simulink model "PTSD_single_channel_local_min_max"  (R2019b)
settings: Solver=VariableStepAuto  StartTime=0.0  StopTime=10  RelTol=1e-3
libraries: simulink x4, dspswit3 x1
settings Model: Creator=sbuccelli  LastModifiedBy=sbuccelli

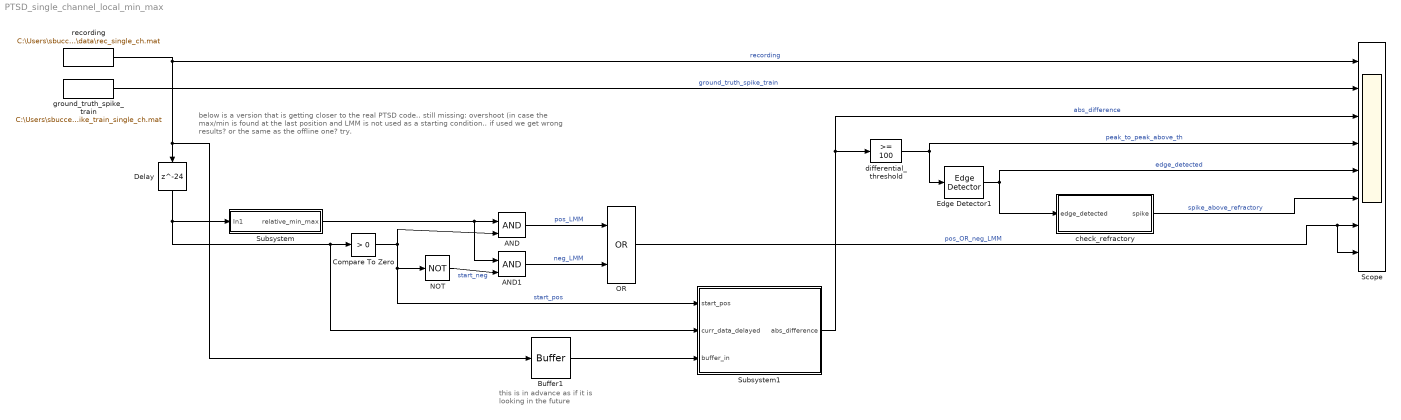
== system PTSD_single_channel_local_min_max ==
  note: below is a version that is getting closer to the real PTSD code..
      | still missing: overshoot (in case the max/min is found at the last position and LMM is not used as a starting condition.. if used we get wrong results? or the same as the offline one? try.
  note: this is in advance as if it is looking in the future
  AND : Logic  IconShape=distinctive  AllPortsSameDT=off  OutDataTypeStr=boolean
  AND1 : Logic  IconShape=distinctive  AllPortsSameDT=off  OutDataTypeStr=boolean
  Buffer1 : Buffer  N=24  V=23  OutputFrames=off
  Compare To Zero : simulink/Logic and Bit Operations/Compare To Zero  relop=>  OutDataTypeStr=boolean
  Delay : Delay  DelayLength=24
  Edge Detector1 : dspswit3/Edge Detector  InputProcessing=Columns as channels (frame based)
      settings: SourceProductName=DSP System Toolbox  SourceProductBaseCode=DS
  NOT : Logic  Operator=NOT  IconShape=distinctive  AllPortsSameDT=off  OutDataTypeStr=boolean
  OR : Logic  Operator=OR  IconShape=distinctive  AllPortsSameDT=off  OutDataTypeStr=boolean
  Scope : Scope  NumInputPorts=8
  Subsystem : Subsystem
  Subsystem1 : Subsystem
  check_refractory : Subsystem
  differential_threshold : simulink/Logic and Bit Operations/Compare To Constant  relop=>=  const=100  OutDataTypeStr=boolean
  ground_truth_spike_train : FromFile  FileName=C:\Users\sbuccelli\Documents\GitHub\closed-loop-neuroscience\data\spike_train_single_ch.mat  SampleTime=1/32e3
  recording : FromFile  FileName=C:\Users\sbuccelli\Documents\GitHub\closed-loop-neuroscience\data\rec_single_ch.mat  SampleTime=1/32e3
  wires:
  recording/1 -> Buffer1/1, Delay/1, Scope/1  "recording"
  ground_truth_spike_train/1 -> Scope/2  "ground_truth_spike_train"
  Subsystem/1(relative_min_max) -> AND/1, AND1/1
  Compare To Zero/1 -> Subsystem1/1(start_pos), NOT/1, AND/2  "start_pos"
  NOT/1 -> AND1/2  "start_neg"
  AND/1 -> OR/1  "pos_LMM"
  AND1/1 -> OR/2  "neg_LMM"
  OR/1 -> Scope/7, Scope/8  "pos_OR_neg_LMM"
  Delay/1 -> Subsystem1/2("curr_data_delayed "), Compare To Zero/1, Subsystem/1(In1)
  differential_threshold/1 -> Scope/4, Edge Detector1/1  "peak_to_peak_above_th"
  Subsystem1/1(abs_difference) -> Scope/3, differential_threshold/1  "abs_difference"
  Buffer1/1 -> Subsystem1/3(buffer_in)
  Edge Detector1/1 -> check_refractory/1(edge_detected), Scope/5  "edge_detected"
  check_refractory/1(spike) -> Scope/6  "spike_above_refractory"

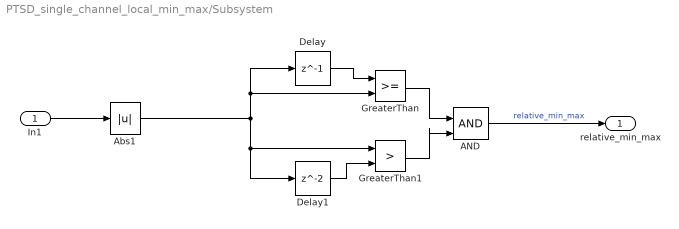
== system PTSD_single_channel_local_min_max/Subsystem ==
  In1 : Inport
  AND : Logic  IconShape=distinctive  AllPortsSameDT=off  OutDataTypeStr=boolean
  Abs1 : Abs
  Delay : Delay  DelayLength=1
  Delay1 : Delay
  GreaterThan : RelationalOperator  OutDataTypeStr=boolean  RndMeth=Simplest
  GreaterThan1 : RelationalOperator  Operator=>  OutDataTypeStr=boolean  RndMeth=Simplest
  relative_min_max : Outport
  wires:
  In1/1 -> Abs1/1
  Delay1/1 -> GreaterThan1/2
  GreaterThan1/1 -> AND/2
  GreaterThan/1 -> AND/1
  Delay/1 -> GreaterThan/1
  AND/1 -> relative_min_max/1  "relative_min_max"
  Abs1/1 -> Delay/1, GreaterThan/2, GreaterThan1/1, Delay1/1

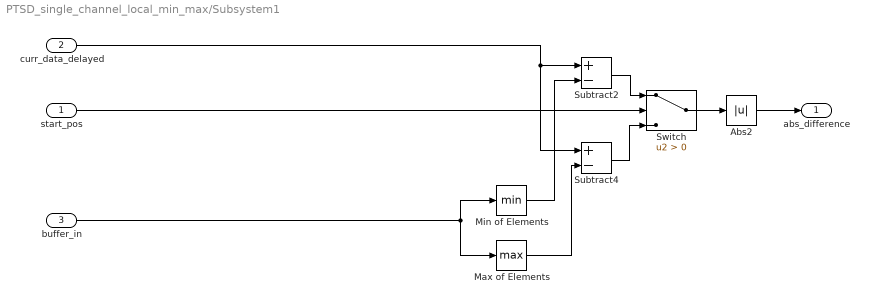
== system PTSD_single_channel_local_min_max/Subsystem1 ==
  start_pos : Inport
  "curr_data_delayed " : Inport  Port=2
  buffer_in : Inport  Port=3
  Abs2 : Abs
  Max of Elements : MinMax  Function=max
  Min of Elements : MinMax
  Subtract2 : Sum  Inputs=+-
  Subtract4 : Sum  Inputs=+-
  Switch : Switch  Criteria=u2 > Threshold
  abs_difference : Outport
  wires:
  Abs2/1 -> abs_difference/1
  buffer_in/1 -> Max of Elements/1, Min of Elements/1
  Switch/1 -> Abs2/1
  Max of Elements/1 -> Subtract4/2
  "curr_data_delayed "/1 -> Subtract4/1, Subtract2/1
  Subtract2/1 -> Switch/1
  Subtract4/1 -> Switch/3
  Min of Elements/1 -> Subtract2/2
  start_pos/1 -> Switch/2

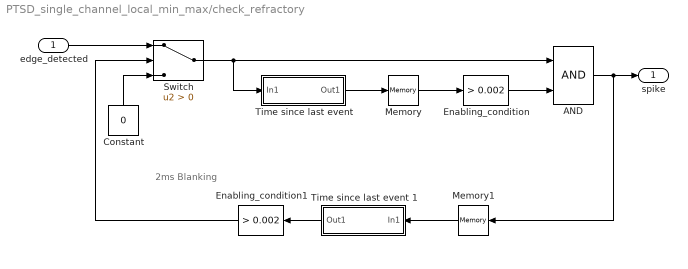
== system PTSD_single_channel_local_min_max/check_refractory ==
  note: 2ms Blanking
  edge_detected : Inport
  AND : Logic  IconShape=distinctive  AllPortsSameDT=off  OutDataTypeStr=boolean
  Constant : Constant  Value=0  SampleTime=-1
  Enabling_condition : simulink/Logic and Bit Operations/Compare To Constant  relop=>  const=0.002  OutDataTypeStr=boolean
  Enabling_condition1 : simulink/Logic and Bit Operations/Compare To Constant  relop=>  const=0.002  OutDataTypeStr=boolean
  Memory : Memory  InheritSampleTime=on
  Memory1 : Memory  InheritSampleTime=on
  Switch : Switch  Criteria=u2 > Threshold
  "Time since last event " : Subsystem
  Time since last event 1 : Subsystem
  spike : Outport
  wires:
  Enabling_condition/1 -> AND/2
  Memory/1 -> Enabling_condition/1
  "Time since last event "/1(Out1) -> Memory/1
  AND/1 -> Memory1/1, spike/1
  Time since last event 1/1(Out1) -> Enabling_condition1/1
  edge_detected/1 -> Switch/1
  Constant/1 -> Switch/3
  Switch/1 -> "Time since last event "/1(In1), AND/1
  Memory1/1 -> Time since last event 1/1(In1)
  Enabling_condition1/1 -> Switch/2

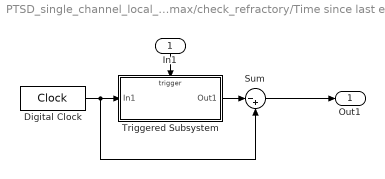
== system PTSD_single_channel_local_min_max/check_refractory/Time since last event  ==
  In1 : Inport
  Digital Clock : DigitalClock  SampleTime=1/32e3
  Sum : Sum  Inputs=|-+
  Triggered Subsystem : Subsystem  TreatAsAtomicUnit=on
  Out1 : Outport
  wires:
  Digital Clock/1 -> Sum/2, Triggered Subsystem/1(In1)
  Triggered Subsystem/1(Out1) -> Sum/1
  In1/1 -> Triggered Subsystem/Trigger
  Sum/1 -> Out1/1

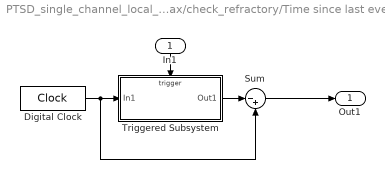
== system PTSD_single_channel_local_min_max/check_refractory/Time since last event 1 ==
  In1 : Inport
  Digital Clock : DigitalClock  SampleTime=1/32e3
  Sum : Sum  Inputs=|-+
  Triggered Subsystem : Subsystem  TreatAsAtomicUnit=on
  Out1 : Outport
  wires:
  Digital Clock/1 -> Sum/2, Triggered Subsystem/1(In1)
  Triggered Subsystem/1(Out1) -> Sum/1
  In1/1 -> Triggered Subsystem/Trigger
  Sum/1 -> Out1/1

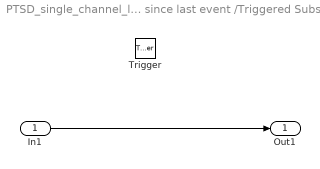
== system PTSD_single_channel_local_min_max/check_refractory/Time since last event /Triggered Subsystem ==
  In1 : Inport
  Trigger : TriggerPort  VariantControl=Variant
  Out1 : Outport
  wires:
  In1/1 -> Out1/1

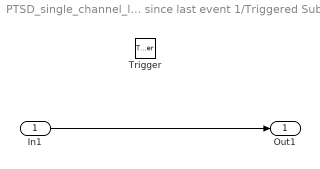
== system PTSD_single_channel_local_min_max/check_refractory/Time since last event 1/Triggered Subsystem ==
  In1 : Inport
  Trigger : TriggerPort  VariantControl=Variant
  Out1 : Outport
  wires:
  In1/1 -> Out1/1
